simulink model "sgMdl_EVSE_ChargeCycleProgression"  (R2024b)
settings: Solver=FixedStepAuto  StartTime=0.0  StopTime=inf  RelTol=1e-3  EnableMultiTasking=on
libraries: speedgoatlib_evse x28
Description:
  | EVSE - Charge Cycle Progression
settings Model: ModifiedByFormat=Speedgoat  SimulationMode=external  ExtModeTrigDuration=100000  Creator=Speedgoat  LastModifiedBy=Speedgoat
settings SolverCC: ConcurrentTasks=on  AlgebraicLoopSolver=TrustRegion  PositivePriorityOrder=on  InsertRTBMode=Never (minimum delay)
settings DataIOCC: SaveFormat=Array  SaveState=on  SignalLoggingName=logsOut
settings OptimizationCC: BlockReduction=off  BooleanDataType=off  OptimizeBlockIOStorage=off  BufferReuse=off  ReuseModelBlockBuffer=off  GlobalBufferReuse=off  ExpressionFolding=off  LocalBlockOutputs=off  InitFltsAndDblsToZero=on  OptimizeDataStoreBuffers=off  BusAssignmentInplaceUpdate=off
settings DebuggingCC: SaveWithParameterizedLinksMsg=none  UnderspecifiedInitializationDetection=Classic  MergeDetectMultiDrivingBlocksExec=none  CheckExecutionContextPreStartOutputMsg=on  SignalResolutionControl=TryResolveAllWithWarning  TasksWithSamePriorityMsg=none  UnconnectedInputMsg=warning  UnconnectedOutputMsg=warning  UnconnectedLineMsg=warning  SFUnexpectedBacktrackingDiag=warning  SFNoUnconditionalDefaultTransitionDiag=warning  SFExecutionAtInitializationDiag=none  ArithmeticOperatorsInVariantConditions=warning
settings HardwareCC: ProdBitPerLong=64  ProdLongLongMode=on  ProdHWDeviceType=Intel->x86-64 (Linux 64)
settings ModelReferenceCC: EnableRefExpFcnMdlSchedulingChecks=on  PropagateSignalLabelsOutOfModel=off
settings SFSimCC: SimUseLocalCustomCode=off  SimTargetLang=C++
settings RTWCC: Description=Speedgoat Real-Time Target Machine  SystemTargetFile=speedgoat.tlc  TemplateMakefile=slrealtime_default_tmf  RTWUseLocalCustomCode=off  Toolchain=Simulink Real-Time Toolchain  BuildConfiguration=Faster Runs  TargetLang=C++  GPUComputeCapability=3.5  DLArmComputeVersion=19.05
settings CodeAppCC: StateflowObjectComments=on
settings SimulinkRealTimeTargetCC: SubcomponentCodeInterfacePackaging=Reusable function  InstructionSetFMA=off  LogToMDFFile=off  SLRTFileLogMaxRuns=10
settings ConfigComp: CovMetricSettings=dw  CovSaveCumulativeToWorkspaceVar=on  CovSaveSingleToWorkspaceVar=on  CovExternalEMLEnable=off  CovSFcnEnable=off  CovBoundaryAbsTol=1.0e-5

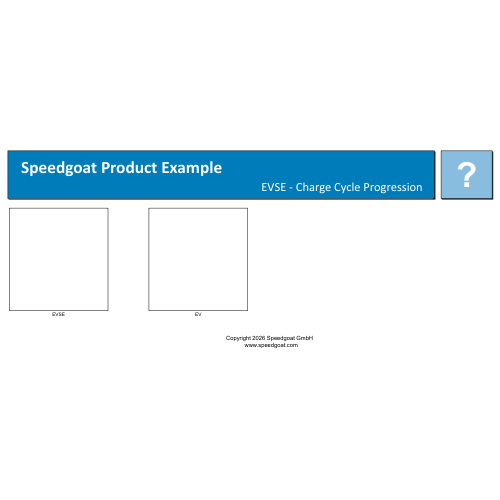
[thumbnail: Simulink's stored preview of the top-level diagram]
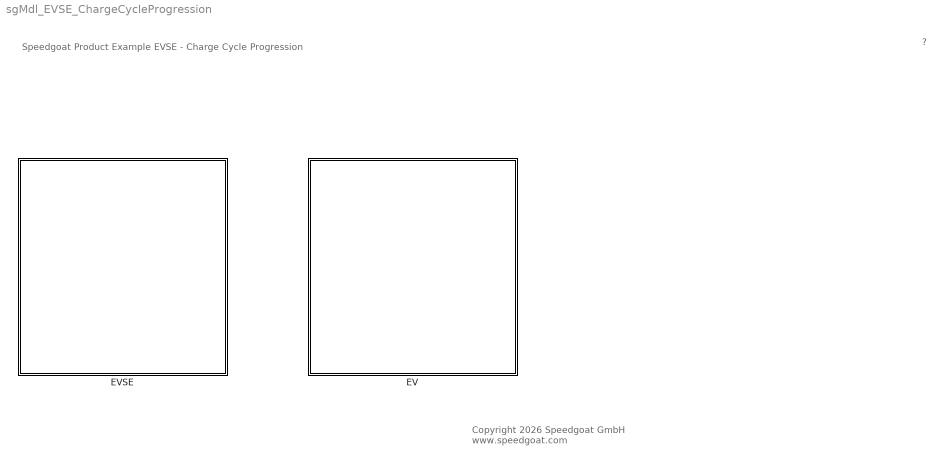
== system sgMdl_EVSE_ChargeCycleProgression ==
  note: Speedgoat Product Example
      | EVSE - Charge Cycle Progression
  note: ?
  note: Copyright 2026 Speedgoat GmbH
      |  www.speedgoat.com
  EV : Subsystem
  EVSE : Subsystem

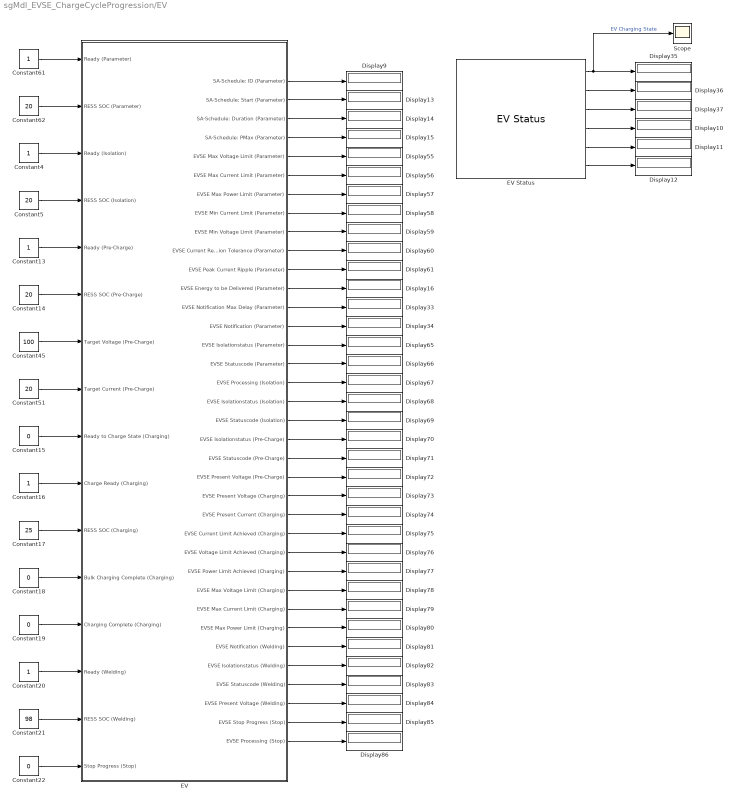
== system sgMdl_EVSE_ChargeCycleProgression/EV ==
  Constant{4,13,16,20,61} (5 alike) : Constant
  Constant{5,14,51,62} (4 alike) : Constant  Value=20
  Constant{15,18..19,22} (4 alike) : Constant  Value=0
  Constant17 : Constant  Value=25
  Constant21 : Constant  Value=98
  Constant45 : Constant  Value=100
  Display{9..16,33..37,55..61,65..86} (42 alike) : Display
  "EV " : Subsystem  mask(EV_EVSE){}
      settings: OpenFcn=sg_evse.openFcnConfig;
      mask Help: eval('sg.utils.help.show(''io_main/refentry_ref_ev_evse'');')
      mask Display: disp('Speedgoat\nEV Charging\nEV\nStation ID: 1');
  "EV Status " : speedgoatlib_evse/EV Status   parClientId=1  parConnectionId=1  parSampleTime=0.1
      settings: SourceProductName=EV Charging
  Scope : Scope
  wires:
  "EV "/25(EVSE Current Limit Achieved (Charging)) -> Display75/1
  "EV "/24(EVSE Present Current (Charging)) -> Display74/1
  "EV "/22(EVSE Present Voltage (Pre-Charge)) -> Display72/1
  "EV "/23(EVSE Present Voltage (Charging)) -> Display73/1
  "EV "/1(SA-Schedule: ID (Parameter)) -> Display9/1
  "EV "/20(EVSE Isolationstatus (Pre-Charge)) -> Display70/1
  Constant45/1 -> "EV "/7(Target Voltage (Pre-Charge))
  Constant61/1 -> "EV "/1(Ready (Parameter))
  "EV "/35(EVSE Stop Progress (Stop)) -> Display85/1
  "EV Status "/5 -> Display11/1
  "EV "/33(EVSE Statuscode (Welding)) -> Display83/1
  "EV "/34(EVSE Present Voltage (Welding)) -> Display84/1
  "EV "/27(EVSE Power Limit Achieved (Charging)) -> Display77/1
  "EV "/26(EVSE Voltage Limit Achieved (Charging)) -> Display76/1
  Constant14/1 -> "EV "/6(RESS SOC (Pre-Charge))
  "EV "/21(EVSE Statuscode (Pre-Charge)) -> Display71/1
  Constant21/1 -> "EV "/15(RESS SOC (Welding))
  "EV "/19(EVSE Statuscode (Isolation)) -> Display69/1
  Constant20/1 -> "EV "/14(Ready (Welding))
  Constant18/1 -> "EV "/12(Bulk Charging Complete (Charging))
  "EV "/10(EVSE Current Regulation Tolerance (Parameter)) -> Display60/1
  "EV "/36(EVSE Processing (Stop)) -> Display86/1
  "EV "/3(SA-Schedule: Duration (Parameter)) -> Display14/1
  "EV "/2(SA-Schedule: Start (Parameter)) -> Display13/1
  Constant13/1 -> "EV "/5(Ready (Pre-Charge))
  Constant17/1 -> "EV "/11(RESS SOC (Charging))
  Constant22/1 -> "EV "/16(Stop Progress (Stop))
  "EV "/29(EVSE Max Current Limit (Charging)) -> Display79/1
  "EV "/17(EVSE Processing (Isolation)) -> Display67/1
  "EV "/28(EVSE Max Voltage Limit (Charging)) -> Display78/1
  "EV Status "/6 -> Display12/1
  Constant15/1 -> "EV "/9(Ready to Charge State (Charging))
  "EV "/16(EVSE Statuscode (Parameter)) -> Display66/1
  Constant62/1 -> "EV "/2(RESS SOC (Parameter))
  "EV "/32(EVSE Isolationstatus (Welding)) -> Display82/1
  Constant4/1 -> "EV "/3(Ready (Isolation))
  "EV "/5(EVSE Max Voltage Limit (Parameter)) -> Display55/1
  "EV "/31(EVSE Notification (Welding)) -> Display81/1
  "EV "/18(EVSE Isolationstatus (Isolation)) -> Display68/1
  "EV "/12(EVSE Energy to be Delivered (Parameter)) -> Display16/1
  Constant5/1 -> "EV "/4(RESS SOC (Isolation))
  "EV "/15(EVSE Isolationstatus (Parameter)) -> Display65/1
  "EV "/11(EVSE Peak Current Ripple (Parameter)) -> Display61/1
  "EV "/13(EVSE Notification Max Delay (Parameter)) -> Display33/1
  "EV "/9(EVSE Min Voltage Limit (Parameter)) -> Display59/1
  "EV "/8(EVSE Min Current Limit (Parameter)) -> Display58/1
  "EV "/14(EVSE Notification (Parameter)) -> Display34/1
  "EV "/7(EVSE Max Power Limit (Parameter)) -> Display57/1
  "EV "/4(SA-Schedule: PMax (Parameter)) -> Display15/1
  "EV Status "/1 -> Scope/1, Display35/1  "EV Charging State"
  "EV "/30(EVSE Max Power Limit (Charging)) -> Display80/1
  "EV Status "/4 -> Display10/1
  Constant16/1 -> "EV "/10(Charge Ready (Charging))
  "EV Status "/3 -> Display37/1
  Constant19/1 -> "EV "/13(Charging Complete (Charging))
  "EV Status "/2 -> Display36/1
  "EV "/6(EVSE Max Current Limit (Parameter)) -> Display56/1
  Constant51/1 -> "EV "/8(Target Current (Pre-Charge))

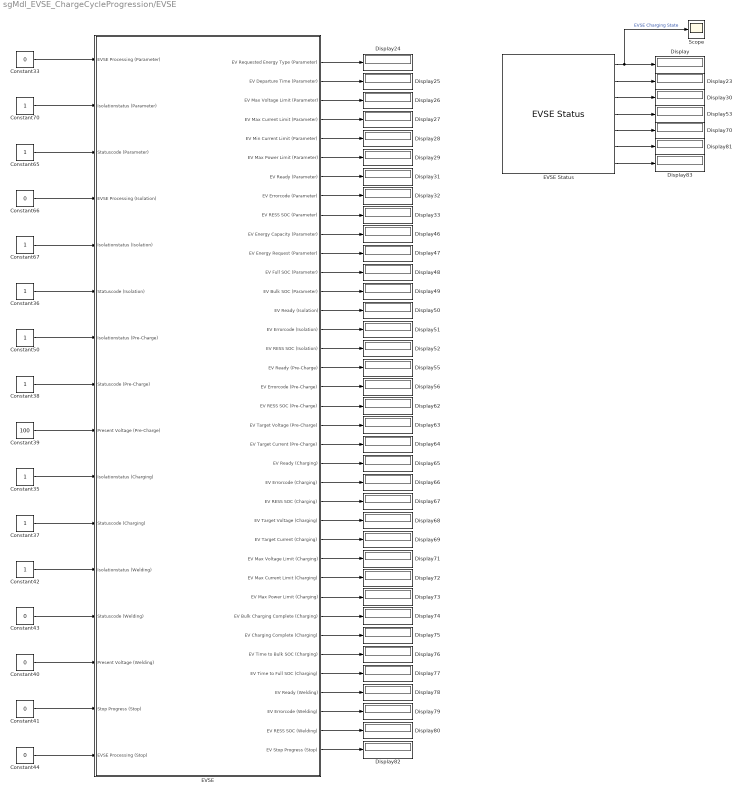
== system sgMdl_EVSE_ChargeCycleProgression/EVSE ==
  Constant{33,40..41,43..44,66} (6 alike) : Constant  Value=0
  Constant{35..38,42,50,65,67,70} (9 alike) : Constant
  Constant39 : Constant  Value=100
  Display{,23..33,46..53,55..56,62..83} (44 alike) : Display
  "EVSE " : Subsystem  mask(EV_EVSE){}
      settings: OpenFcn=sg_evse.openFcnConfig;
      mask Help: eval('sg.utils.help.show(''io_main/refentry_ref_ev_evse'');')
      mask Display: disp('Speedgoat\nEV Charging\nEVSE\nStation ID: 0');
  "EVSE Status " : speedgoatlib_evse/EVSE Status   parClientId=0  parConnectionId=0  parSampleTime=0.1
      settings: SourceProductName=EV Charging
  Scope : Scope
  wires:
  Constant44/1 -> "EVSE "/16(EVSE Processing (Stop))
  "EVSE "/36(EV RESS SOC (Welding)) -> Display80/1
  "EVSE Status "/5 -> Display70/1
  Constant66/1 -> "EVSE "/4(EVSE Processing (Isolation))
  Constant42/1 -> "EVSE "/12(Isolationstatus (Welding))
  Constant67/1 -> "EVSE "/5(Isolationstatus (Isolation))
  Constant41/1 -> "EVSE "/15(Stop Progress (Stop))
  Constant39/1 -> "EVSE "/9(Present Voltage (Pre-Charge))
  Constant40/1 -> "EVSE "/14(Present Voltage (Welding))
  "EVSE "/37(EV Stop Progress (Stop)) -> Display82/1
  "EVSE Status "/7 -> Display83/1
  "EVSE "/27(EV Max Voltage Limit (Charging)) -> Display71/1
  "EVSE "/3(EV Max Voltage Limit (Parameter)) -> Display26/1
  Constant70/1 -> "EVSE "/2(Isolationstatus (Parameter))
  "EVSE "/10(EV Energy Capacity (Parameter)) -> Display46/1
  "EVSE "/32(EV Time to Bulk SOC (Charging)) -> Display76/1
  "EVSE "/5(EV Min Current Limit (Parameter)) -> Display28/1
  "EVSE Status "/1 -> Scope/1, Display/1  "EVSE Charging State"
  "EVSE Status "/2 -> Display23/1
  "EVSE "/21(EV Target Current (Pre-Charge)) -> Display64/1
  Constant36/1 -> "EVSE "/6(Statuscode (Isolation))
  "EVSE "/17(EV Ready (Pre-Charge)) -> Display55/1
  Constant33/1 -> "EVSE "/1(EVSE Processing (Parameter))
  "EVSE "/33(EV Time to Full SOC (Charging)) -> Display77/1
  "EVSE "/29(EV Max Power Limit (Charging)) -> Display73/1
  "EVSE "/18(EV Errorcode (Pre-Charge)) -> Display56/1
  "EVSE "/31(EV Charging Complete (Charging)) -> Display75/1
  Constant65/1 -> "EVSE "/3(Statuscode (Parameter))
  "EVSE "/19(EV RESS SOC (Pre-Charge)) -> Display62/1
  Constant43/1 -> "EVSE "/13(Statuscode (Welding))
  "EVSE "/14(EV Ready (Isolation)) -> Display50/1
  "EVSE "/26(EV Target Current (Charging)) -> Display69/1
  "EVSE "/34(EV Ready (Welding)) -> Display78/1
  "EVSE Status "/4 -> Display53/1
  "EVSE "/30(EV Bulk Charging Complete (Charging)) -> Display74/1
  "EVSE "/24(EV RESS SOC (Charging)) -> Display67/1
  "EVSE "/22(EV Ready (Charging)) -> Display65/1
  "EVSE "/23(EV Errorcode (Charging)) -> Display66/1
  "EVSE "/15(EV Errorcode (Isolation)) -> Display51/1
  "EVSE "/12(EV Full SOC (Parameter)) -> Display48/1
  "EVSE "/7(EV Ready (Parameter)) -> Display31/1
  Constant37/1 -> "EVSE "/11(Statuscode (Charging))
  Constant50/1 -> "EVSE "/7(Isolationstatus (Pre-Charge))
  "EVSE "/13(EV Bulk SOC (Parameter)) -> Display49/1
  "EVSE "/16(EV RESS SOC (Isolation)) -> Display52/1
  "EVSE "/9(EV RESS SOC (Parameter)) -> Display33/1
  Constant38/1 -> "EVSE "/8(Statuscode (Pre-Charge))
  "EVSE "/1(EV Requested Energy Type (Parameter)) -> Display24/1
  "EVSE "/28(EV Max Current Limit (Charging)) -> Display72/1
  "EVSE "/20(EV Target Voltage (Pre-Charge)) -> Display63/1
  "EVSE "/4(EV Max Current Limit (Parameter)) -> Display27/1
  "EVSE "/35(EV Errorcode (Welding)) -> Display79/1
  "EVSE "/2(EV Departure Time (Parameter)) -> Display25/1
  "EVSE "/8(EV Errorcode (Parameter)) -> Display32/1
  "EVSE Status "/3 -> Display30/1
  Constant35/1 -> "EVSE "/10(Isolationstatus (Charging))
  "EVSE Status "/6 -> Display81/1
  "EVSE "/6(EV Max Power Limit (Parameter)) -> Display29/1
  "EVSE "/11(EV Energy Request (Parameter)) -> Display47/1
  "EVSE "/25(EV Target Voltage (Charging)) -> Display68/1

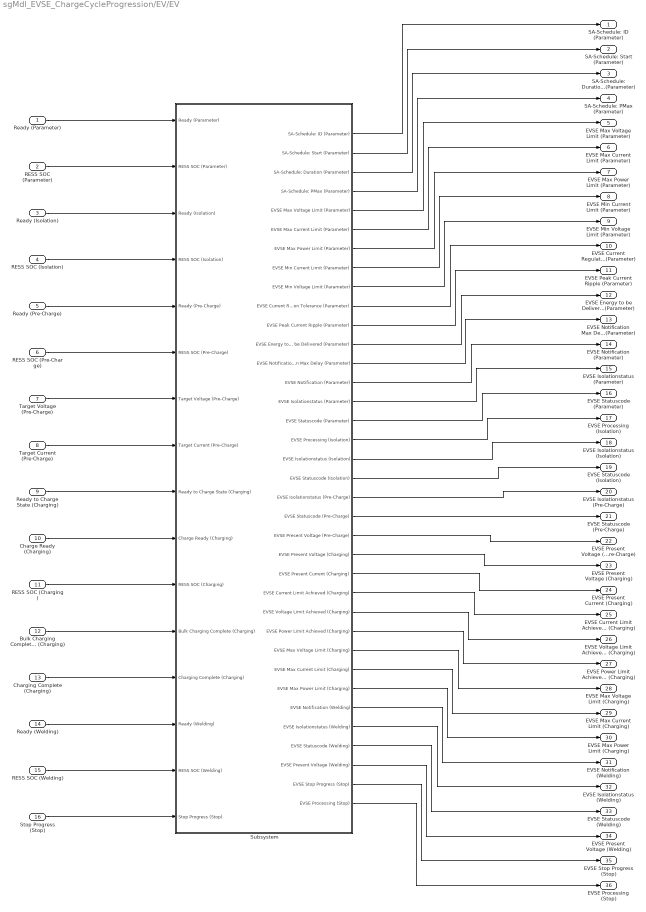
== system sgMdl_EVSE_ChargeCycleProgression/EV/EV  ==
  Ready (Parameter) : Inport
  RESS SOC (Parameter) : Inport  Port=2
  Ready (Isolation) : Inport  Port=3
  RESS SOC (Isolation) : Inport  Port=4
  Ready (Pre-Charge) : Inport  Port=5
  RESS SOC (Pre-Charge) : Inport  Port=6
  Target Voltage (Pre-Charge) : Inport  Port=7
  Target Current (Pre-Charge) : Inport  Port=8
  Ready to Charge State (Charging) : Inport  Port=9
  Charge Ready (Charging) : Inport  Port=10
  RESS SOC (Charging) : Inport  Port=11
  Bulk Charging Complete (Charging) : Inport  Port=12
  Charging Complete (Charging) : Inport  Port=13
  Ready (Welding) : Inport  Port=14
  RESS SOC (Welding) : Inport  Port=15
  Stop Progress (Stop) : Inport  Port=16
  Subsystem : Subsystem
  SA-Schedule: ID (Parameter) : Outport
  SA-Schedule: Start (Parameter) : Outport  Port=2
  SA-Schedule: Duration (Parameter) : Outport  Port=3
  SA-Schedule: PMax (Parameter) : Outport  Port=4
  EVSE Max Voltage Limit (Parameter) : Outport  Port=5
  EVSE Max Current Limit (Parameter) : Outport  Port=6
  EVSE Max Power Limit (Parameter) : Outport  Port=7
  EVSE Min Current Limit (Parameter) : Outport  Port=8
  EVSE Min Voltage Limit (Parameter) : Outport  Port=9
  EVSE Current Regulation Tolerance (Parameter) : Outport  Port=10
  EVSE Peak Current Ripple (Parameter) : Outport  Port=11
  EVSE Energy to be Delivered (Parameter) : Outport  Port=12
  EVSE Notification Max Delay (Parameter) : Outport  Port=13
  EVSE Notification (Parameter) : Outport  Port=14
  EVSE Isolationstatus (Parameter) : Outport  Port=15
  EVSE Statuscode (Parameter) : Outport  Port=16
  EVSE Processing (Isolation) : Outport  Port=17
  EVSE Isolationstatus (Isolation) : Outport  Port=18
  EVSE Statuscode (Isolation) : Outport  Port=19
  EVSE Isolationstatus (Pre-Charge) : Outport  Port=20
  EVSE Statuscode (Pre-Charge) : Outport  Port=21
  EVSE Present Voltage (Pre-Charge) : Outport  Port=22
  EVSE Present Voltage (Charging) : Outport  Port=23
  EVSE Present Current (Charging) : Outport  Port=24
  EVSE Current Limit Achieved (Charging) : Outport  Port=25
  EVSE Voltage Limit Achieved (Charging) : Outport  Port=26
  EVSE Power Limit Achieved (Charging) : Outport  Port=27
  EVSE Max Voltage Limit (Charging) : Outport  Port=28
  EVSE Max Current Limit (Charging) : Outport  Port=29
  EVSE Max Power Limit (Charging) : Outport  Port=30
  EVSE Notification (Welding) : Outport  Port=31
  EVSE Isolationstatus (Welding) : Outport  Port=32
  EVSE Statuscode (Welding) : Outport  Port=33
  EVSE Present Voltage (Welding) : Outport  Port=34
  EVSE Stop Progress (Stop) : Outport  Port=35
  EVSE Processing (Stop) : Outport  Port=36
  wires:
  Subsystem/20(EVSE Isolationstatus (Pre-Charge)) -> EVSE Isolationstatus (Pre-Charge)/1
  RESS SOC (Parameter)/1 -> Subsystem/2(RESS SOC (Parameter))
  RESS SOC (Isolation)/1 -> Subsystem/4(RESS SOC (Isolation))
  Ready (Parameter)/1 -> Subsystem/1(Ready (Parameter))
  Ready (Isolation)/1 -> Subsystem/3(Ready (Isolation))
  Subsystem/6(EVSE Max Current Limit (Parameter)) -> EVSE Max Current Limit (Parameter)/1
  Bulk Charging Complete (Charging)/1 -> Subsystem/12(Bulk Charging Complete (Charging))
  Charge Ready (Charging)/1 -> Subsystem/10(Charge Ready (Charging))
  RESS SOC (Pre-Charge)/1 -> Subsystem/6(RESS SOC (Pre-Charge))
  Target Current (Pre-Charge)/1 -> Subsystem/8(Target Current (Pre-Charge))
  RESS SOC (Charging)/1 -> Subsystem/11(RESS SOC (Charging))
  Ready to Charge State (Charging)/1 -> Subsystem/9(Ready to Charge State (Charging))
  Ready (Pre-Charge)/1 -> Subsystem/5(Ready (Pre-Charge))
  Target Voltage (Pre-Charge)/1 -> Subsystem/7(Target Voltage (Pre-Charge))
  Subsystem/12(EVSE Energy to be Delivered (Parameter)) -> EVSE Energy to be Delivered (Parameter)/1
  RESS SOC (Welding)/1 -> Subsystem/15(RESS SOC (Welding))
  Charging Complete (Charging)/1 -> Subsystem/13(Charging Complete (Charging))
  Subsystem/32(EVSE Isolationstatus (Welding)) -> EVSE Isolationstatus (Welding)/1
  Stop Progress (Stop)/1 -> Subsystem/16(Stop Progress (Stop))
  Ready (Welding)/1 -> Subsystem/14(Ready (Welding))
  Subsystem/1(SA-Schedule: ID (Parameter)) -> SA-Schedule: ID (Parameter)/1
  Subsystem/2(SA-Schedule: Start (Parameter)) -> SA-Schedule: Start (Parameter)/1
  Subsystem/3(SA-Schedule: Duration (Parameter)) -> SA-Schedule: Duration (Parameter)/1
  Subsystem/36(EVSE Processing (Stop)) -> EVSE Processing (Stop)/1
  Subsystem/4(SA-Schedule: PMax (Parameter)) -> SA-Schedule: PMax (Parameter)/1
  Subsystem/5(EVSE Max Voltage Limit (Parameter)) -> EVSE Max Voltage Limit (Parameter)/1
  Subsystem/7(EVSE Max Power Limit (Parameter)) -> EVSE Max Power Limit (Parameter)/1
  Subsystem/8(EVSE Min Current Limit (Parameter)) -> EVSE Min Current Limit (Parameter)/1
  Subsystem/9(EVSE Min Voltage Limit (Parameter)) -> EVSE Min Voltage Limit (Parameter)/1
  Subsystem/10(EVSE Current Regulation Tolerance (Parameter)) -> EVSE Current Regulation Tolerance (Parameter)/1
  Subsystem/11(EVSE Peak Current Ripple (Parameter)) -> EVSE Peak Current Ripple (Parameter)/1
  Subsystem/13(EVSE Notification Max Delay (Parameter)) -> EVSE Notification Max Delay (Parameter)/1
  Subsystem/24(EVSE Present Current (Charging)) -> EVSE Present Current (Charging)/1
  Subsystem/14(EVSE Notification (Parameter)) -> EVSE Notification (Parameter)/1
  Subsystem/15(EVSE Isolationstatus (Parameter)) -> EVSE Isolationstatus (Parameter)/1
  Subsystem/26(EVSE Voltage Limit Achieved (Charging)) -> EVSE Voltage Limit Achieved (Charging)/1
  Subsystem/16(EVSE Statuscode (Parameter)) -> EVSE Statuscode (Parameter)/1
  Subsystem/17(EVSE Processing (Isolation)) -> EVSE Processing (Isolation)/1
  Subsystem/18(EVSE Isolationstatus (Isolation)) -> EVSE Isolationstatus (Isolation)/1
  Subsystem/19(EVSE Statuscode (Isolation)) -> EVSE Statuscode (Isolation)/1
  Subsystem/21(EVSE Statuscode (Pre-Charge)) -> EVSE Statuscode (Pre-Charge)/1
  Subsystem/22(EVSE Present Voltage (Pre-Charge)) -> EVSE Present Voltage (Pre-Charge)/1
  Subsystem/23(EVSE Present Voltage (Charging)) -> EVSE Present Voltage (Charging)/1
  Subsystem/25(EVSE Current Limit Achieved (Charging)) -> EVSE Current Limit Achieved (Charging)/1
  Subsystem/27(EVSE Power Limit Achieved (Charging)) -> EVSE Power Limit Achieved (Charging)/1
  Subsystem/28(EVSE Max Voltage Limit (Charging)) -> EVSE Max Voltage Limit (Charging)/1
  Subsystem/29(EVSE Max Current Limit (Charging)) -> EVSE Max Current Limit (Charging)/1
  Subsystem/30(EVSE Max Power Limit (Charging)) -> EVSE Max Power Limit (Charging)/1
  Subsystem/31(EVSE Notification (Welding)) -> EVSE Notification (Welding)/1
  Subsystem/33(EVSE Statuscode (Welding)) -> EVSE Statuscode (Welding)/1
  Subsystem/34(EVSE Present Voltage (Welding)) -> EVSE Present Voltage (Welding)/1
  Subsystem/35(EVSE Stop Progress (Stop)) -> EVSE Stop Progress (Stop)/1

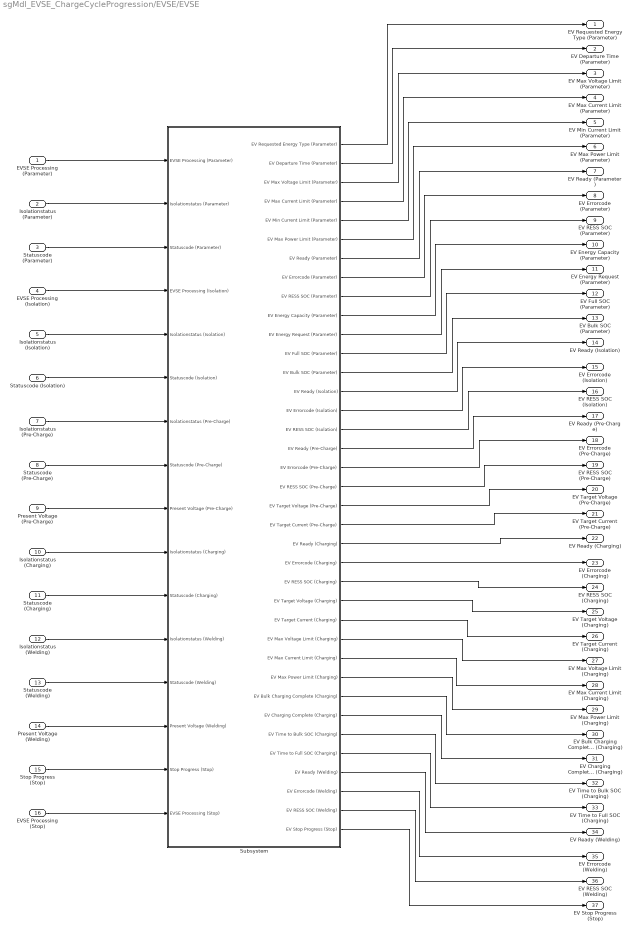
== system sgMdl_EVSE_ChargeCycleProgression/EVSE/EVSE  ==
  EVSE Processing (Parameter) : Inport
  Isolationstatus (Parameter) : Inport  Port=2
  Statuscode (Parameter) : Inport  Port=3
  EVSE Processing (Isolation) : Inport  Port=4
  Isolationstatus (Isolation) : Inport  Port=5
  Statuscode (Isolation) : Inport  Port=6
  Isolationstatus (Pre-Charge) : Inport  Port=7
  Statuscode (Pre-Charge) : Inport  Port=8
  Present Voltage (Pre-Charge) : Inport  Port=9
  Isolationstatus (Charging) : Inport  Port=10
  Statuscode (Charging) : Inport  Port=11
  Isolationstatus (Welding) : Inport  Port=12
  Statuscode (Welding) : Inport  Port=13
  Present Voltage (Welding) : Inport  Port=14
  Stop Progress (Stop) : Inport  Port=15
  EVSE Processing (Stop) : Inport  Port=16
  Subsystem : Subsystem
  EV Requested Energy Type (Parameter) : Outport
  EV Departure Time (Parameter) : Outport  Port=2
  EV Max Voltage Limit (Parameter) : Outport  Port=3
  EV Max Current Limit (Parameter) : Outport  Port=4
  EV Min Current Limit (Parameter) : Outport  Port=5
  EV Max Power Limit (Parameter) : Outport  Port=6
  EV Ready (Parameter) : Outport  Port=7
  EV Errorcode (Parameter) : Outport  Port=8
  EV RESS SOC (Parameter) : Outport  Port=9
  EV Energy Capacity (Parameter) : Outport  Port=10
  EV Energy Request (Parameter) : Outport  Port=11
  EV Full SOC (Parameter) : Outport  Port=12
  EV Bulk SOC (Parameter) : Outport  Port=13
  EV Ready (Isolation) : Outport  Port=14
  EV Errorcode (Isolation) : Outport  Port=15
  EV RESS SOC (Isolation) : Outport  Port=16
  EV Ready (Pre-Charge) : Outport  Port=17
  EV Errorcode (Pre-Charge) : Outport  Port=18
  EV RESS SOC (Pre-Charge) : Outport  Port=19
  EV Target Voltage (Pre-Charge) : Outport  Port=20
  EV Target Current (Pre-Charge) : Outport  Port=21
  EV Ready (Charging) : Outport  Port=22
  EV Errorcode (Charging) : Outport  Port=23
  EV RESS SOC (Charging) : Outport  Port=24
  EV Target Voltage (Charging) : Outport  Port=25
  EV Target Current (Charging) : Outport  Port=26
  EV Max Voltage Limit (Charging) : Outport  Port=27
  EV Max Current Limit (Charging) : Outport  Port=28
  EV Max Power Limit (Charging) : Outport  Port=29
  EV Bulk Charging Complete (Charging) : Outport  Port=30
  EV Charging Complete (Charging) : Outport  Port=31
  EV Time to Bulk SOC (Charging) : Outport  Port=32
  EV Time to Full SOC (Charging) : Outport  Port=33
  EV Ready (Welding) : Outport  Port=34
  EV Errorcode (Welding) : Outport  Port=35
  EV RESS SOC (Welding) : Outport  Port=36
  EV Stop Progress (Stop) : Outport  Port=37
  wires:
  Isolationstatus (Isolation)/1 -> Subsystem/5(Isolationstatus (Isolation))
  Subsystem/35(EV Errorcode (Welding)) -> EV Errorcode (Welding)/1
  EVSE Processing (Isolation)/1 -> Subsystem/4(EVSE Processing (Isolation))
  Statuscode (Parameter)/1 -> Subsystem/3(Statuscode (Parameter))
  Subsystem/26(EV Target Current (Charging)) -> EV Target Current (Charging)/1
  Isolationstatus (Parameter)/1 -> Subsystem/2(Isolationstatus (Parameter))
  EVSE Processing (Parameter)/1 -> Subsystem/1(EVSE Processing (Parameter))
  EVSE Processing (Stop)/1 -> Subsystem/16(EVSE Processing (Stop))
  Statuscode (Pre-Charge)/1 -> Subsystem/8(Statuscode (Pre-Charge))
  Subsystem/36(EV RESS SOC (Welding)) -> EV RESS SOC (Welding)/1
  Subsystem/2(EV Departure Time (Parameter)) -> EV Departure Time (Parameter)/1
  Stop Progress (Stop)/1 -> Subsystem/15(Stop Progress (Stop))
  Isolationstatus (Pre-Charge)/1 -> Subsystem/7(Isolationstatus (Pre-Charge))
  Subsystem/9(EV RESS SOC (Parameter)) -> EV RESS SOC (Parameter)/1
  Present Voltage (Welding)/1 -> Subsystem/14(Present Voltage (Welding))
  Statuscode (Isolation)/1 -> Subsystem/6(Statuscode (Isolation))
  Present Voltage (Pre-Charge)/1 -> Subsystem/9(Present Voltage (Pre-Charge))
  Isolationstatus (Charging)/1 -> Subsystem/10(Isolationstatus (Charging))
  Statuscode (Charging)/1 -> Subsystem/11(Statuscode (Charging))
  Subsystem/33(EV Time to Full SOC (Charging)) -> EV Time to Full SOC (Charging)/1
  Isolationstatus (Welding)/1 -> Subsystem/12(Isolationstatus (Welding))
  Subsystem/27(EV Max Voltage Limit (Charging)) -> EV Max Voltage Limit (Charging)/1
  Statuscode (Welding)/1 -> Subsystem/13(Statuscode (Welding))
  Subsystem/1(EV Requested Energy Type (Parameter)) -> EV Requested Energy Type (Parameter)/1
  Subsystem/3(EV Max Voltage Limit (Parameter)) -> EV Max Voltage Limit (Parameter)/1
  Subsystem/4(EV Max Current Limit (Parameter)) -> EV Max Current Limit (Parameter)/1
  Subsystem/5(EV Min Current Limit (Parameter)) -> EV Min Current Limit (Parameter)/1
  Subsystem/6(EV Max Power Limit (Parameter)) -> EV Max Power Limit (Parameter)/1
  Subsystem/7(EV Ready (Parameter)) -> EV Ready (Parameter)/1
  Subsystem/8(EV Errorcode (Parameter)) -> EV Errorcode (Parameter)/1
  Subsystem/10(EV Energy Capacity (Parameter)) -> EV Energy Capacity (Parameter)/1
  Subsystem/11(EV Energy Request (Parameter)) -> EV Energy Request (Parameter)/1
  Subsystem/12(EV Full SOC (Parameter)) -> EV Full SOC (Parameter)/1
  Subsystem/13(EV Bulk SOC (Parameter)) -> EV Bulk SOC (Parameter)/1
  Subsystem/14(EV Ready (Isolation)) -> EV Ready (Isolation)/1
  Subsystem/15(EV Errorcode (Isolation)) -> EV Errorcode (Isolation)/1
  Subsystem/16(EV RESS SOC (Isolation)) -> EV RESS SOC (Isolation)/1
  Subsystem/17(EV Ready (Pre-Charge)) -> EV Ready (Pre-Charge)/1
  Subsystem/18(EV Errorcode (Pre-Charge)) -> EV Errorcode (Pre-Charge)/1
  Subsystem/19(EV RESS SOC (Pre-Charge)) -> EV RESS SOC (Pre-Charge)/1
  Subsystem/20(EV Target Voltage (Pre-Charge)) -> EV Target Voltage (Pre-Charge)/1
  Subsystem/21(EV Target Current (Pre-Charge)) -> EV Target Current (Pre-Charge)/1
  Subsystem/22(EV Ready (Charging)) -> EV Ready (Charging)/1
  Subsystem/23(EV Errorcode (Charging)) -> EV Errorcode (Charging)/1
  Subsystem/24(EV RESS SOC (Charging)) -> EV RESS SOC (Charging)/1
  Subsystem/25(EV Target Voltage (Charging)) -> EV Target Voltage (Charging)/1
  Subsystem/28(EV Max Current Limit (Charging)) -> EV Max Current Limit (Charging)/1
  Subsystem/29(EV Max Power Limit (Charging)) -> EV Max Power Limit (Charging)/1
  Subsystem/30(EV Bulk Charging Complete (Charging)) -> EV Bulk Charging Complete (Charging)/1
  Subsystem/31(EV Charging Complete (Charging)) -> EV Charging Complete (Charging)/1
  Subsystem/32(EV Time to Bulk SOC (Charging)) -> EV Time to Bulk SOC (Charging)/1
  Subsystem/34(EV Ready (Welding)) -> EV Ready (Welding)/1
  Subsystem/37(EV Stop Progress (Stop)) -> EV Stop Progress (Stop)/1

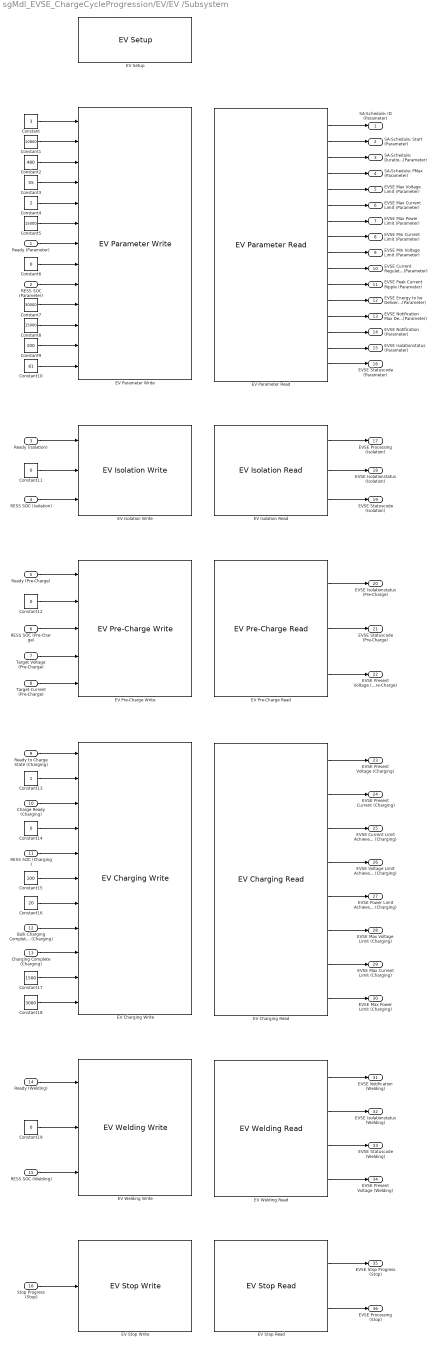
== system sgMdl_EVSE_ChargeCycleProgression/EV/EV /Subsystem ==
  Ready (Parameter) : Inport
  RESS SOC (Parameter) : Inport  Port=2
  Ready (Isolation) : Inport  Port=3
  RESS SOC (Isolation) : Inport  Port=4
  Ready (Pre-Charge) : Inport  Port=5
  RESS SOC (Pre-Charge) : Inport  Port=6
  Target Voltage (Pre-Charge) : Inport  Port=7
  Target Current (Pre-Charge) : Inport  Port=8
  Ready to Charge State (Charging) : Inport  Port=9
  Charge Ready (Charging) : Inport  Port=10
  RESS SOC (Charging) : Inport  Port=11
  Bulk Charging Complete (Charging) : Inport  Port=12
  Charging Complete (Charging) : Inport  Port=13
  Ready (Welding) : Inport  Port=14
  RESS SOC (Welding) : Inport  Port=15
  Stop Progress (Stop) : Inport  Port=16
  Constant : Constant  Value=3
  Constant1 : Constant  Value=10800
  Constant10 : Constant  Value=81
  Constant{6,11..12,14,19} (5 alike) : Constant  Value=0
  Constant13 : Constant
  Constant15 : Constant  Value=100
  Constant16 : Constant  Value=20
  Constant17 : Constant  Value=1500
  Constant18 : Constant  Value=3000
  Constant2 : Constant  Value=480
  Constant3 : Constant  Value=55
  Constant4 : Constant  Value=2
  Constant5 : Constant  Value=15000
  Constant7 : Constant  Value=30000
  Constant8 : Constant  Value=15000
  Constant9 : Constant  Value=100
  "EV Charging Read " : speedgoatlib_evse/Blocks by Charge State/EV Charging Read   parClientId=1  parConnectionId=1  parSampleTime=0.1
      settings: SourceProductName=EV Charging
  "EV Charging Write " : speedgoatlib_evse/Blocks by Charge State/EV Charging Write   parClientId=1  parConnectionId=1  parSampleTime=0.1  parEnReadyToChargeState=on  parEnChargingProfileTupleId=on  parEnChargeReady=on  parEnErrorCode=on  parEnRessSoc=on  parEnTargetVoltage=on  parEnTargetCurrent=on  parEnBulkChargingComplete=on  parEnChargingComplete=on  parEnRemainingTimeToBulkSoc=on  parEnRemainingTimeToFullSoc=on
      settings: SourceProductName=EV Charging
  "EV Isolation Read " : speedgoatlib_evse/Blocks by Charge State/EV Isolation Read   parClientId=1  parConnectionId=1  parSampleTime=0.1
      settings: SourceProductName=EV Charging
  "EV Isolation Write " : speedgoatlib_evse/Blocks by Charge State/EV Isolation Write   parClientId=1  parConnectionId=1  parSampleTime=0.1  parEnReady=on  parEnErrorCode=on  parEnRessSoc=on
      settings: SourceProductName=EV Charging
  "EV Parameter Read " : speedgoatlib_evse/Blocks by Charge State/EV Parameter Read   parClientId=1  parConnectionId=1  parSampleTime=0.1
      settings: SourceProductName=EV Charging
  "EV Parameter Write " : speedgoatlib_evse/Blocks by Charge State/EV Parameter Write   parClientId=1  parConnectionId=1  parSampleTime=0.1  parEnRequestedEnergyType=on  parEnDepartureTime=on  parEnMaxVoltageLimit=on  parEnMaxCurrentLimit=on  parEnMinCurrentLimit=on  parEnMaxPowerLimit=on  parEnReady=on  parEnErrorcode=on  parEnRessSoc=on  parEnEnergyCapacity=on  parEnEnergyRequest=on  parEnFullSoc=on  parEnBulkSoc=on
      settings: SourceProductName=EV Charging
  "EV Pre-Charge Read " : speedgoatlib_evse/Blocks by Charge State/EV Pre-Charge Read   parClientId=1  parConnectionId=1  parSampleTime=0.1
      settings: SourceProductName=EV Charging
  "EV Pre-Charge Write " : speedgoatlib_evse/Blocks by Charge State/EV Pre-Charge Write   parClientId=1  parConnectionId=1  parSampleTime=0.1  parEnReady=on  parEnErrorCode=on  parEnRessSoc=on  parEnTargetVoltage=on  parEnTargetCurrent=on
      settings: SourceProductName=EV Charging
  "EV Setup " : speedgoatlib_evse/Blocks by Charge State/EV Setup   parClientId=1  parConnectionId=1  parClientIdentifier='speedgoat'  parIpAddrStr='169.254.12.50'  parSampleTime=0.1  parTcpPort=1883  parRemoteIpAddrStr='169.254.12.53'  parDepartureTime=14400  parMaxVoltageLimit=480  parMaxCurrentLimit=100  parMinCurrentLimit=5  parMaxPowerLimit=60000  parRessSoc=30  parEnergyCapacity=80000  parEnergyRequest=30000  parFullSoc=100  parBulkSoc=80
      settings: SourceProductName=EV Charging
  "EV Stop Read " : speedgoatlib_evse/Blocks by Charge State/EV Stop Read   parClientId=1  parConnectionId=1  parSampleTime=0.1
      settings: SourceProductName=EV Charging
  "EV Stop Write " : speedgoatlib_evse/Blocks by Charge State/EV Stop Write   parClientId=1  parConnectionId=1  parSampleTime=0.1  parEnStopProgress=on
      settings: SourceProductName=EV Charging
  "EV Welding Read " : speedgoatlib_evse/Blocks by Charge State/EV Welding Read   parClientId=1  parConnectionId=1  parSampleTime=0.1
      settings: SourceProductName=EV Charging
  "EV Welding Write " : speedgoatlib_evse/Blocks by Charge State/EV Welding Write   parClientId=1  parConnectionId=1  parSampleTime=0.1  parEnReady=on  parEnErrorCode=on  parEnRessSoc=on
      settings: SourceProductName=EV Charging
  SA-Schedule: ID (Parameter) : Outport
  SA-Schedule: Start (Parameter) : Outport  Port=2
  SA-Schedule: Duration (Parameter) : Outport  Port=3
  SA-Schedule: PMax (Parameter) : Outport  Port=4
  EVSE Max Voltage Limit (Parameter) : Outport  Port=5
  EVSE Max Current Limit (Parameter) : Outport  Port=6
  EVSE Max Power Limit (Parameter) : Outport  Port=7
  EVSE Min Current Limit (Parameter) : Outport  Port=8
  EVSE Min Voltage Limit (Parameter) : Outport  Port=9
  EVSE Current Regulation Tolerance (Parameter) : Outport  Port=10
  EVSE Peak Current Ripple (Parameter) : Outport  Port=11
  EVSE Energy to be Delivered (Parameter) : Outport  Port=12
  EVSE Notification Max Delay (Parameter) : Outport  Port=13
  EVSE Notification (Parameter) : Outport  Port=14
  EVSE Isolationstatus (Parameter) : Outport  Port=15
  EVSE Statuscode (Parameter) : Outport  Port=16
  EVSE Processing (Isolation) : Outport  Port=17
  EVSE Isolationstatus (Isolation) : Outport  Port=18
  EVSE Statuscode (Isolation) : Outport  Port=19
  EVSE Isolationstatus (Pre-Charge) : Outport  Port=20
  EVSE Statuscode (Pre-Charge) : Outport  Port=21
  EVSE Present Voltage (Pre-Charge) : Outport  Port=22
  EVSE Present Voltage (Charging) : Outport  Port=23
  EVSE Present Current (Charging) : Outport  Port=24
  EVSE Current Limit Achieved (Charging) : Outport  Port=25
  EVSE Voltage Limit Achieved (Charging) : Outport  Port=26
  EVSE Power Limit Achieved (Charging) : Outport  Port=27
  EVSE Max Voltage Limit (Charging) : Outport  Port=28
  EVSE Max Current Limit (Charging) : Outport  Port=29
  EVSE Max Power Limit (Charging) : Outport  Port=30
  EVSE Notification (Welding) : Outport  Port=31
  EVSE Isolationstatus (Welding) : Outport  Port=32
  EVSE Statuscode (Welding) : Outport  Port=33
  EVSE Present Voltage (Welding) : Outport  Port=34
  EVSE Stop Progress (Stop) : Outport  Port=35
  EVSE Processing (Stop) : Outport  Port=36
  wires:
  Constant/1 -> "EV Parameter Write "/1
  Constant1/1 -> "EV Parameter Write "/2
  Constant2/1 -> "EV Parameter Write "/3
  Constant3/1 -> "EV Parameter Write "/4
  Constant4/1 -> "EV Parameter Write "/5
  Constant5/1 -> "EV Parameter Write "/6
  Ready (Parameter)/1 -> "EV Parameter Write "/7
  Constant6/1 -> "EV Parameter Write "/8
  RESS SOC (Parameter)/1 -> "EV Parameter Write "/9
  Constant7/1 -> "EV Parameter Write "/10
  Constant8/1 -> "EV Parameter Write "/11
  Constant9/1 -> "EV Parameter Write "/12
  Constant10/1 -> "EV Parameter Write "/13
  "EV Parameter Read "/1 -> SA-Schedule: ID (Parameter)/1
  "EV Parameter Read "/2 -> SA-Schedule: Start (Parameter)/1
  "EV Parameter Read "/3 -> SA-Schedule: Duration (Parameter)/1
  "EV Parameter Read "/4 -> SA-Schedule: PMax (Parameter)/1
  "EV Parameter Read "/5 -> EVSE Max Voltage Limit (Parameter)/1
  "EV Parameter Read "/6 -> EVSE Max Current Limit (Parameter)/1
  "EV Parameter Read "/7 -> EVSE Max Power Limit (Parameter)/1
  "EV Parameter Read "/8 -> EVSE Min Current Limit (Parameter)/1
  "EV Parameter Read "/9 -> EVSE Min Voltage Limit (Parameter)/1
  "EV Parameter Read "/10 -> EVSE Current Regulation Tolerance (Parameter)/1
  "EV Parameter Read "/11 -> EVSE Peak Current Ripple (Parameter)/1
  "EV Parameter Read "/12 -> EVSE Energy to be Delivered (Parameter)/1
  "EV Parameter Read "/13 -> EVSE Notification Max Delay (Parameter)/1
  "EV Parameter Read "/14 -> EVSE Notification (Parameter)/1
  "EV Parameter Read "/15 -> EVSE Isolationstatus (Parameter)/1
  "EV Parameter Read "/16 -> EVSE Statuscode (Parameter)/1
  Ready (Isolation)/1 -> "EV Isolation Write "/1
  Constant11/1 -> "EV Isolation Write "/2
  RESS SOC (Isolation)/1 -> "EV Isolation Write "/3
  "EV Isolation Read "/1 -> EVSE Processing (Isolation)/1
  "EV Isolation Read "/2 -> EVSE Isolationstatus (Isolation)/1
  "EV Isolation Read "/3 -> EVSE Statuscode (Isolation)/1
  Ready (Pre-Charge)/1 -> "EV Pre-Charge Write "/1
  Constant12/1 -> "EV Pre-Charge Write "/2
  RESS SOC (Pre-Charge)/1 -> "EV Pre-Charge Write "/3
  Target Voltage (Pre-Charge)/1 -> "EV Pre-Charge Write "/4
  Target Current (Pre-Charge)/1 -> "EV Pre-Charge Write "/5
  "EV Pre-Charge Read "/1 -> EVSE Isolationstatus (Pre-Charge)/1
  "EV Pre-Charge Read "/2 -> EVSE Statuscode (Pre-Charge)/1
  "EV Pre-Charge Read "/3 -> EVSE Present Voltage (Pre-Charge)/1
  Ready to Charge State (Charging)/1 -> "EV Charging Write "/1
  Constant13/1 -> "EV Charging Write "/2
  Charge Ready (Charging)/1 -> "EV Charging Write "/3
  Constant14/1 -> "EV Charging Write "/4
  RESS SOC (Charging)/1 -> "EV Charging Write "/5
  Constant15/1 -> "EV Charging Write "/6
  Constant16/1 -> "EV Charging Write "/7
  Bulk Charging Complete (Charging)/1 -> "EV Charging Write "/8
  Charging Complete (Charging)/1 -> "EV Charging Write "/9
  Constant17/1 -> "EV Charging Write "/10
  Constant18/1 -> "EV Charging Write "/11
  "EV Charging Read "/1 -> EVSE Present Voltage (Charging)/1
  "EV Charging Read "/2 -> EVSE Present Current (Charging)/1
  "EV Charging Read "/3 -> EVSE Current Limit Achieved (Charging)/1
  "EV Charging Read "/4 -> EVSE Voltage Limit Achieved (Charging)/1
  "EV Charging Read "/5 -> EVSE Power Limit Achieved (Charging)/1
  "EV Charging Read "/6 -> EVSE Max Voltage Limit (Charging)/1
  "EV Charging Read "/7 -> EVSE Max Current Limit (Charging)/1
  "EV Charging Read "/8 -> EVSE Max Power Limit (Charging)/1
  Ready (Welding)/1 -> "EV Welding Write "/1
  Constant19/1 -> "EV Welding Write "/2
  RESS SOC (Welding)/1 -> "EV Welding Write "/3
  "EV Welding Read "/1 -> EVSE Notification (Welding)/1
  "EV Welding Read "/2 -> EVSE Isolationstatus (Welding)/1
  "EV Welding Read "/3 -> EVSE Statuscode (Welding)/1
  "EV Welding Read "/4 -> EVSE Present Voltage (Welding)/1
  Stop Progress (Stop)/1 -> "EV Stop Write "/1
  "EV Stop Read "/1 -> EVSE Stop Progress (Stop)/1
  "EV Stop Read "/2 -> EVSE Processing (Stop)/1

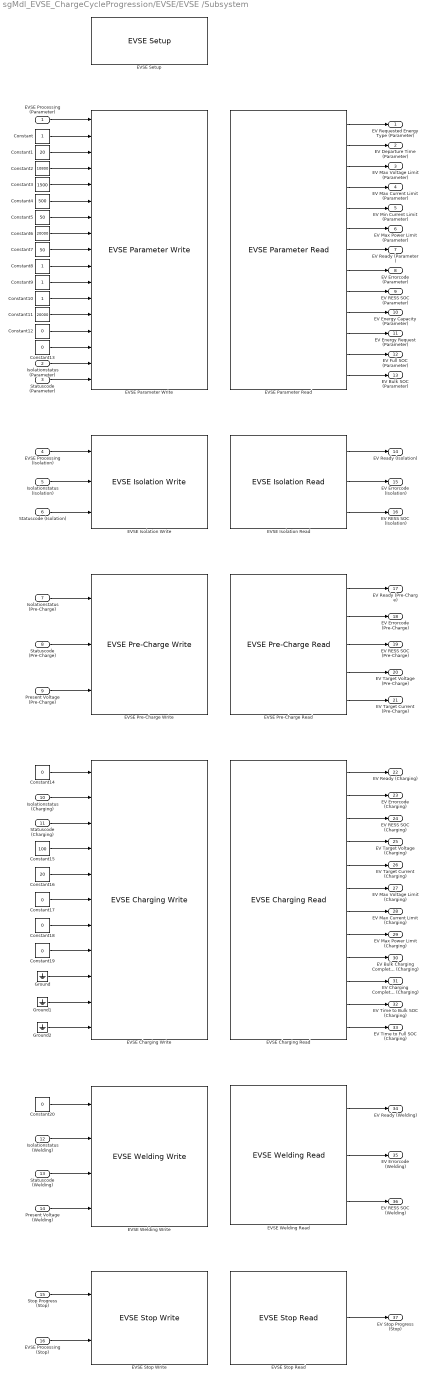
== system sgMdl_EVSE_ChargeCycleProgression/EVSE/EVSE /Subsystem ==
  EVSE Processing (Parameter) : Inport
  Isolationstatus (Parameter) : Inport  Port=2
  Statuscode (Parameter) : Inport  Port=3
  EVSE Processing (Isolation) : Inport  Port=4
  Isolationstatus (Isolation) : Inport  Port=5
  Statuscode (Isolation) : Inport  Port=6
  Isolationstatus (Pre-Charge) : Inport  Port=7
  Statuscode (Pre-Charge) : Inport  Port=8
  Present Voltage (Pre-Charge) : Inport  Port=9
  Isolationstatus (Charging) : Inport  Port=10
  Statuscode (Charging) : Inport  Port=11
  Isolationstatus (Welding) : Inport  Port=12
  Statuscode (Welding) : Inport  Port=13
  Present Voltage (Welding) : Inport  Port=14
  Stop Progress (Stop) : Inport  Port=15
  EVSE Processing (Stop) : Inport  Port=16
  Constant{,8..10} (4 alike) : Constant
  Constant1 : Constant  Value=20
  Constant11 : Constant  Value=20000
  Constant{12..14,17..20} (7 alike) : Constant  Value=0
  Constant15 : Constant  Value=100
  Constant16 : Constant  Value=20
  Constant2 : Constant  Value=10800
  Constant3 : Constant  Value=1500
  Constant4 : Constant  Value=500
  Constant5 : Constant  Value=50
  Constant6 : Constant  Value=20000
  Constant7 : Constant  Value=50
  "EVSE Charging Read " : speedgoatlib_evse/Blocks by Charge State/EVSE Charging Read   parClientId=0  parConnectionId=0  parSampleTime=0.1
      settings: SourceProductName=EV Charging
  "EVSE Charging Write " : speedgoatlib_evse/Blocks by Charge State/EVSE Charging Write   parClientId=0  parConnectionId=0  parSampleTime=0.1  parEnNotification=on  parEnIsolationStatus=on  parEnStatusCode=on  parEnPresentVoltage=on  parEnPresentCurrent=on  parEnCurrentLimitAchieved=on  parEnVoltageLimitAchieved=on  parEnPowerLimitAchieved=on  parEnMaxVoltageLimit=off  parEnMaxCurrentLimit=off  parEnMaxPowerLimit=off
      settings: SourceProductName=EV Charging
  "EVSE Isolation Read " : speedgoatlib_evse/Blocks by Charge State/EVSE Isolation Read   parClientId=0  parConnectionId=0  parSampleTime=0.1
      settings: SourceProductName=EV Charging
  "EVSE Isolation Write " : speedgoatlib_evse/Blocks by Charge State/EVSE Isolation Write   parClientId=0  parConnectionId=0  parSampleTime=0.1  parEnEvseProcessing=on  parEnIsolationStatus=on  parEnStatusCode=on
      settings: SourceProductName=EV Charging
  "EVSE Parameter Read " : speedgoatlib_evse/Blocks by Charge State/EVSE Parameter Read   parClientId=0  parConnectionId=0  parSampleTime=0.1
      settings: SourceProductName=EV Charging
  "EVSE Parameter Write " : speedgoatlib_evse/Blocks by Charge State/EVSE Parameter Write   parClientId=0  parConnectionId=0  parSampleTime=0.1  parEnEvseProcessing=on  parEnSaScheduleList=on  parEnMaxVoltageLimit=on  parEnMaxCurrentLimit=on  parEnMaxPowerLimit=on  parEnMinVoltageLimit=on  parEnMinCurrentLimit=on  parEnCurrRegTol=on  parEnPeakCurrentRipple=on  parEnEnergyToBeDelivered=on  parEnNotificationMaxDelay=on  parEnNotification=on  parEnIsolationStatus=on  parEnStatusCode=on
      settings: SourceProductName=EV Charging
  "EVSE Pre-Charge Read " : speedgoatlib_evse/Blocks by Charge State/EVSE Pre-Charge Read   parClientId=0  parConnectionId=0  parSampleTime=0.1
      settings: SourceProductName=EV Charging
  "EVSE Pre-Charge Write " : speedgoatlib_evse/Blocks by Charge State/EVSE Pre-Charge Write   parClientId=0  parConnectionId=0  parSampleTime=0.1  parEnIsolationStatus=on  parEnStatusCode=on  parEnPresentVoltage=on
      settings: SourceProductName=EV Charging
  "EVSE Setup " : speedgoatlib_evse/Blocks by Charge State/EVSE Setup   parClientId=0  parConnectionId=0  parClientIdentifier='speedgoat'  parIpAddrStr='169.254.12.50'  parSampleTime=0.1  parTcpPort=1883  parRemoteIpAddrStr='169.254.12.53'  parMaxVoltageLimit=480  parMaxCurrentLimit=100  parMinCurrentLimit=0  parMaxPowerLimit=60000  parMinVoltageLimit=12  parCurrRegTol=5  parPeakCurrentRipple=0
      settings: SourceProductName=EV Charging
  "EVSE Stop Read " : speedgoatlib_evse/Blocks by Charge State/EVSE Stop Read   parClientId=0  parConnectionId=0  parSampleTime=0.1
      settings: SourceProductName=EV Charging
  "EVSE Stop Write " : speedgoatlib_evse/Blocks by Charge State/EVSE Stop Write   parClientId=0  parConnectionId=0  parSampleTime=0.1  parEnStopProgress=on  parEnEvseProcessing=on
      settings: SourceProductName=EV Charging
  "EVSE Welding Read " : speedgoatlib_evse/Blocks by Charge State/EVSE Welding Read   parClientId=0  parConnectionId=0  parSampleTime=0.1
      settings: SourceProductName=EV Charging
  "EVSE Welding Write " : speedgoatlib_evse/Blocks by Charge State/EVSE Welding Write   parClientId=0  parConnectionId=0  parSampleTime=0.1  parEnNotification=on  parEnIsolationStatus=on  parEnStatusCode=on  parEnPresentVoltage=on
      settings: SourceProductName=EV Charging
  Ground : Ground
  Ground1 : Ground
  Ground2 : Ground
  EV Requested Energy Type (Parameter) : Outport
  EV Departure Time (Parameter) : Outport  Port=2
  EV Max Voltage Limit (Parameter) : Outport  Port=3
  EV Max Current Limit (Parameter) : Outport  Port=4
  EV Min Current Limit (Parameter) : Outport  Port=5
  EV Max Power Limit (Parameter) : Outport  Port=6
  EV Ready (Parameter) : Outport  Port=7
  EV Errorcode (Parameter) : Outport  Port=8
  EV RESS SOC (Parameter) : Outport  Port=9
  EV Energy Capacity (Parameter) : Outport  Port=10
  EV Energy Request (Parameter) : Outport  Port=11
  EV Full SOC (Parameter) : Outport  Port=12
  EV Bulk SOC (Parameter) : Outport  Port=13
  EV Ready (Isolation) : Outport  Port=14
  EV Errorcode (Isolation) : Outport  Port=15
  EV RESS SOC (Isolation) : Outport  Port=16
  EV Ready (Pre-Charge) : Outport  Port=17
  EV Errorcode (Pre-Charge) : Outport  Port=18
  EV RESS SOC (Pre-Charge) : Outport  Port=19
  EV Target Voltage (Pre-Charge) : Outport  Port=20
  EV Target Current (Pre-Charge) : Outport  Port=21
  EV Ready (Charging) : Outport  Port=22
  EV Errorcode (Charging) : Outport  Port=23
  EV RESS SOC (Charging) : Outport  Port=24
  EV Target Voltage (Charging) : Outport  Port=25
  EV Target Current (Charging) : Outport  Port=26
  EV Max Voltage Limit (Charging) : Outport  Port=27
  EV Max Current Limit (Charging) : Outport  Port=28
  EV Max Power Limit (Charging) : Outport  Port=29
  EV Bulk Charging Complete (Charging) : Outport  Port=30
  EV Charging Complete (Charging) : Outport  Port=31
  EV Time to Bulk SOC (Charging) : Outport  Port=32
  EV Time to Full SOC (Charging) : Outport  Port=33
  EV Ready (Welding) : Outport  Port=34
  EV Errorcode (Welding) : Outport  Port=35
  EV RESS SOC (Welding) : Outport  Port=36
  EV Stop Progress (Stop) : Outport  Port=37
  wires:
  EVSE Processing (Parameter)/1 -> "EVSE Parameter Write "/1
  Constant/1 -> "EVSE Parameter Write "/2
  Constant1/1 -> "EVSE Parameter Write "/3
  Constant2/1 -> "EVSE Parameter Write "/4
  Constant3/1 -> "EVSE Parameter Write "/5
  Constant4/1 -> "EVSE Parameter Write "/6
  Constant5/1 -> "EVSE Parameter Write "/7
  Constant6/1 -> "EVSE Parameter Write "/8
  Constant7/1 -> "EVSE Parameter Write "/9
  Constant8/1 -> "EVSE Parameter Write "/10
  Constant9/1 -> "EVSE Parameter Write "/11
  Constant10/1 -> "EVSE Parameter Write "/12
  Constant11/1 -> "EVSE Parameter Write "/13
  Constant12/1 -> "EVSE Parameter Write "/14
  Constant13/1 -> "EVSE Parameter Write "/15
  Isolationstatus (Parameter)/1 -> "EVSE Parameter Write "/16
  Statuscode (Parameter)/1 -> "EVSE Parameter Write "/17
  "EVSE Parameter Read "/1 -> EV Requested Energy Type (Parameter)/1
  "EVSE Parameter Read "/2 -> EV Departure Time (Parameter)/1
  "EVSE Parameter Read "/3 -> EV Max Voltage Limit (Parameter)/1
  "EVSE Parameter Read "/4 -> EV Max Current Limit (Parameter)/1
  "EVSE Parameter Read "/5 -> EV Min Current Limit (Parameter)/1
  "EVSE Parameter Read "/6 -> EV Max Power Limit (Parameter)/1
  "EVSE Parameter Read "/7 -> EV Ready (Parameter)/1
  "EVSE Parameter Read "/8 -> EV Errorcode (Parameter)/1
  "EVSE Parameter Read "/9 -> EV RESS SOC (Parameter)/1
  "EVSE Parameter Read "/10 -> EV Energy Capacity (Parameter)/1
  "EVSE Parameter Read "/11 -> EV Energy Request (Parameter)/1
  "EVSE Parameter Read "/12 -> EV Full SOC (Parameter)/1
  "EVSE Parameter Read "/13 -> EV Bulk SOC (Parameter)/1
  EVSE Processing (Isolation)/1 -> "EVSE Isolation Write "/1
  Isolationstatus (Isolation)/1 -> "EVSE Isolation Write "/2
  Statuscode (Isolation)/1 -> "EVSE Isolation Write "/3
  "EVSE Isolation Read "/1 -> EV Ready (Isolation)/1
  "EVSE Isolation Read "/2 -> EV Errorcode (Isolation)/1
  "EVSE Isolation Read "/3 -> EV RESS SOC (Isolation)/1
  Isolationstatus (Pre-Charge)/1 -> "EVSE Pre-Charge Write "/1
  Statuscode (Pre-Charge)/1 -> "EVSE Pre-Charge Write "/2
  Present Voltage (Pre-Charge)/1 -> "EVSE Pre-Charge Write "/3
  "EVSE Pre-Charge Read "/1 -> EV Ready (Pre-Charge)/1
  "EVSE Pre-Charge Read "/2 -> EV Errorcode (Pre-Charge)/1
  "EVSE Pre-Charge Read "/3 -> EV RESS SOC (Pre-Charge)/1
  "EVSE Pre-Charge Read "/4 -> EV Target Voltage (Pre-Charge)/1
  "EVSE Pre-Charge Read "/5 -> EV Target Current (Pre-Charge)/1
  Constant14/1 -> "EVSE Charging Write "/1
  Isolationstatus (Charging)/1 -> "EVSE Charging Write "/2
  Statuscode (Charging)/1 -> "EVSE Charging Write "/3
  Constant15/1 -> "EVSE Charging Write "/4
  Constant16/1 -> "EVSE Charging Write "/5
  Constant17/1 -> "EVSE Charging Write "/6
  Constant18/1 -> "EVSE Charging Write "/7
  Constant19/1 -> "EVSE Charging Write "/8
  Ground/1 -> "EVSE Charging Write "/9
  Ground1/1 -> "EVSE Charging Write "/10
  Ground2/1 -> "EVSE Charging Write "/11
  "EVSE Charging Read "/1 -> EV Ready (Charging)/1
  "EVSE Charging Read "/2 -> EV Errorcode (Charging)/1
  "EVSE Charging Read "/3 -> EV RESS SOC (Charging)/1
  "EVSE Charging Read "/4 -> EV Target Voltage (Charging)/1
  "EVSE Charging Read "/5 -> EV Target Current (Charging)/1
  "EVSE Charging Read "/6 -> EV Max Voltage Limit (Charging)/1
  "EVSE Charging Read "/7 -> EV Max Current Limit (Charging)/1
  "EVSE Charging Read "/8 -> EV Max Power Limit (Charging)/1
  "EVSE Charging Read "/9 -> EV Bulk Charging Complete (Charging)/1
  "EVSE Charging Read "/10 -> EV Charging Complete (Charging)/1
  "EVSE Charging Read "/11 -> EV Time to Bulk SOC (Charging)/1
  "EVSE Charging Read "/12 -> EV Time to Full SOC (Charging)/1
  Constant20/1 -> "EVSE Welding Write "/1
  Isolationstatus (Welding)/1 -> "EVSE Welding Write "/2
  Statuscode (Welding)/1 -> "EVSE Welding Write "/3
  Present Voltage (Welding)/1 -> "EVSE Welding Write "/4
  "EVSE Welding Read "/1 -> EV Ready (Welding)/1
  "EVSE Welding Read "/2 -> EV Errorcode (Welding)/1
  "EVSE Welding Read "/3 -> EV RESS SOC (Welding)/1
  Stop Progress (Stop)/1 -> "EVSE Stop Write "/1
  EVSE Processing (Stop)/1 -> "EVSE Stop Write "/2
  "EVSE Stop Read "/1 -> EV Stop Progress (Stop)/1
